simulink model "DSQPID"  (Simulink 7.8)
settings: Solver=ode4  StartTime=0.0  StopTime=2  FixedStep=0.001  RelTol=1e-3
settings Model: Creator=Zhu Supeng  LastModifiedBy=Zhu Supeng
settings DataIOCC: SignalLoggingName=sigsOut
settings DebuggingCC: SaveWithParameterizedLinksMsg=none  SignalResolutionControl=TryResolveAllWithWarning  SolverPrmCheckMsg=none  MultiTaskDSMMsg=warning  MultiTaskCondExecSysMsg=none  StrictBusMsg=None
settings HardwareCC: TargetUnknown=on
settings RTWCC: IncludeERTFirstTime=on

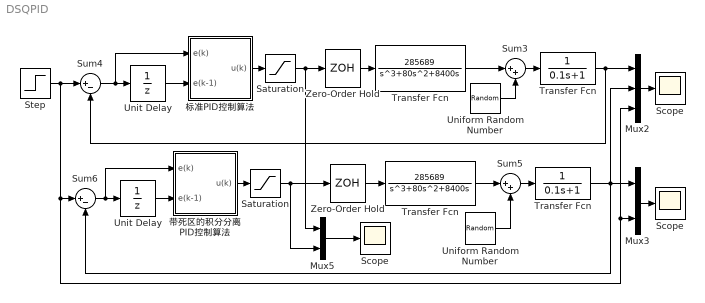
== system DSQPID ==
  "  Transfer Fcn " : TransferFcn  Denominator=[0.1 1]
  " Transfer Fcn " : TransferFcn  Denominator=[0.1 1]
  Mux2 : Mux  Inputs=3
  Mux3 : Mux  Inputs=2
  Mux5 : Mux  Inputs=2
  Saturation : Saturate  UpperLimit=10  LowerLimit=-10
  "Saturation " : Saturate  UpperLimit=10  LowerLimit=-10
  Scope : Scope
      settings: YMin=0.955  YMax=1.035  SaveName=DSQPIDy  DataFormat=Array  MaxDataPoints=500000
  "Scope " : Scope
      settings: YMin=-2  YMax=10  SaveName=DSQPIDu  DataFormat=Array  MaxDataPoints=500000
  "Scope  " : Scope
      settings: YMin=-0.2  YMax=1.2  SaveName=DSQPIDry  DataFormat=Array  MaxDataPoints=500000
  Step : Step  Time=0  SampleTime=0
  Sum3 : Sum  Inputs=|++  SaturateOnIntegerOverflow=on
  Sum4 : Sum  Inputs=|+-  SaturateOnIntegerOverflow=on
  Sum5 : Sum  Inputs=|++  SaturateOnIntegerOverflow=on
  Sum6 : Sum  Inputs=|+-  SaturateOnIntegerOverflow=on
  Transfer Fcn : TransferFcn  Numerator=[285689]  Denominator=[1 80 8400 0]
  "Transfer Fcn " : TransferFcn  Numerator=[285689]  Denominator=[1 80 8400 0]
  "Uniform Random Number " : UniformRandomNumber  Minimum=-0.5  Maximum=0.5  SampleTime=0
  "Uniform Random Number   " : UniformRandomNumber  Minimum=-0.5  Maximum=0.5  SampleTime=0
  Unit Delay : UnitDelay  SampleTime=0.001
  "Unit Delay " : UnitDelay  SampleTime=0.001
  Zero-Order Hold : ZeroOrderHold  SampleTime=0.001
  "Zero-Order Hold " : ZeroOrderHold  SampleTime=0.001
  带死区的积分分离 PID控制算法 : Subsystem
  标准PID控制算法 : Subsystem
  wires:
  "Transfer Fcn "/1 -> Sum5/1
  Sum5/1 -> " Transfer Fcn "/1
  "Uniform Random Number "/1 -> Sum5/2
  带死区的积分分离 PID控制算法/1(u(k)) -> "Saturation "/1
  "Unit Delay "/1 -> 带死区的积分分离 PID控制算法/2(e(k-1))
  Mux3/1 -> Scope/1
  " Transfer Fcn "/1 -> Mux3/1, Mux2/2, Sum6/2
  "Zero-Order Hold "/1 -> "Transfer Fcn "/1
  Mux5/1 -> "Scope "/1
  Step/1 -> Sum6/1, Mux2/3, Mux3/2, Sum4/1
  "Saturation "/1 -> "Zero-Order Hold "/1, Mux5/2
  Sum6/1 -> "Unit Delay "/1, 带死区的积分分离 PID控制算法/1(e(k))
  Transfer Fcn/1 -> Sum3/1
  Sum3/1 -> "  Transfer Fcn "/1
  标准PID控制算法/1(u(k)) -> Saturation/1
  Unit Delay/1 -> 标准PID控制算法/2(e(k-1))
  Sum4/1 -> 标准PID控制算法/1(e(k)), Unit Delay/1
  Mux2/1 -> "Scope  "/1
  Zero-Order Hold/1 -> Transfer Fcn/1
  Saturation/1 -> Zero-Order Hold/1, Mux5/1
  "  Transfer Fcn "/1 -> Sum4/2, Mux2/1
  "Uniform Random Number   "/1 -> Sum3/2

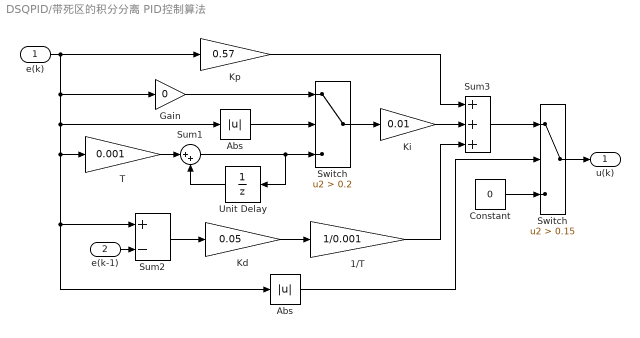
== system DSQPID/带死区的积分分离 PID控制算法 ==
  e(k) : Inport
  e(k-1) : Inport  Port=2
  1/T : Gain  Gain=1/0.001  SaturateOnIntegerOverflow=on  OutDataTypeStr=Inherit: Same as input  ParamDataTypeStr=Inherit: Same as input
  Abs : Abs  SaturateOnIntegerOverflow=on
  "Abs " : Abs  SaturateOnIntegerOverflow=on
  Constant : Constant  Value=0
  Gain : Gain  Gain=0  SaturateOnIntegerOverflow=on  OutDataTypeStr=Inherit: Same as input  ParamDataTypeStr=Inherit: Same as input
  Kd : Gain  Gain=0.05  SaturateOnIntegerOverflow=on  OutDataTypeStr=Inherit: Same as input  ParamDataTypeStr=Inherit: Same as input
  Ki : Gain  Gain=0.01  SaturateOnIntegerOverflow=on  OutDataTypeStr=Inherit: Same as input  ParamDataTypeStr=Inherit: Same as input
  Kp : Gain  Gain=0.57  SaturateOnIntegerOverflow=on  OutDataTypeStr=Inherit: Same as input  ParamDataTypeStr=Inherit: Same as input
  Sum1 : Sum  Inputs=|++  SaturateOnIntegerOverflow=on
  Sum2 : Sum  Inputs=+-  SaturateOnIntegerOverflow=on
  Sum3 : Sum  Inputs=+++  SaturateOnIntegerOverflow=on
  Switch : Switch  Criteria=u2 > Threshold  Threshold=0.2  SaturateOnIntegerOverflow=on  InputSameDT=on
  "Switch " : Switch  Criteria=u2 > Threshold  Threshold=0.15  SaturateOnIntegerOverflow=on  InputSameDT=on
  T : Gain  Gain=0.001  SaturateOnIntegerOverflow=on  OutDataTypeStr=Inherit: Same as input  ParamDataTypeStr=Inherit: Same as input
  "Unit Delay " : UnitDelay  SampleTime=0.001
  u(k) : Outport
  wires:
  Sum3/1 -> "Switch "/1
  Ki/1 -> Sum3/2
  1/T/1 -> Sum3/3
  e(k-1)/1 -> Sum2/2
  Kd/1 -> 1/T/1
  Kp/1 -> Sum3/1
  e(k)/1 -> Kp/1, Gain/1, Abs/1, T/1, Sum2/1, "Abs "/1
  Sum2/1 -> Kd/1
  T/1 -> Sum1/1
  "Unit Delay "/1 -> Sum1/2
  Sum1/1 -> "Unit Delay "/1, Switch/3
  "Abs "/1 -> "Switch "/2
  Constant/1 -> "Switch "/3
  "Switch "/1 -> u(k)/1
  Switch/1 -> Ki/1
  Gain/1 -> Switch/1
  Abs/1 -> Switch/2

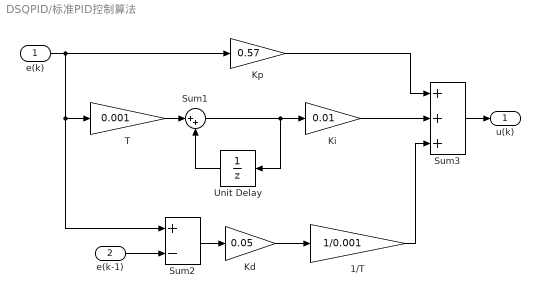
== system DSQPID/标准PID控制算法 ==
  e(k) : Inport
  e(k-1) : Inport  Port=2
  1/T : Gain  Gain=1/0.001  SaturateOnIntegerOverflow=on  OutDataTypeStr=Inherit: Same as input  ParamDataTypeStr=Inherit: Same as input
  Kd : Gain  Gain=0.05  SaturateOnIntegerOverflow=on  OutDataTypeStr=Inherit: Same as input  ParamDataTypeStr=Inherit: Same as input
  Ki : Gain  Gain=0.01  SaturateOnIntegerOverflow=on  OutDataTypeStr=Inherit: Same as input  ParamDataTypeStr=Inherit: Same as input
  Kp : Gain  Gain=0.57  SaturateOnIntegerOverflow=on  OutDataTypeStr=Inherit: Same as input  ParamDataTypeStr=Inherit: Same as input
  Sum1 : Sum  Inputs=|++  SaturateOnIntegerOverflow=on
  Sum2 : Sum  Inputs=+-  SaturateOnIntegerOverflow=on
  Sum3 : Sum  Inputs=+++  SaturateOnIntegerOverflow=on
  T : Gain  Gain=0.001  SaturateOnIntegerOverflow=on  OutDataTypeStr=Inherit: Same as input  ParamDataTypeStr=Inherit: Same as input
  Unit Delay : UnitDelay  SampleTime=0.001
  u(k) : Outport
  wires:
  Sum3/1 -> u(k)/1
  Ki/1 -> Sum3/2
  1/T/1 -> Sum3/3
  e(k-1)/1 -> Sum2/2
  Kd/1 -> 1/T/1
  Kp/1 -> Sum3/1
  e(k)/1 -> Kp/1, Sum2/1, T/1
  Sum2/1 -> Kd/1
  T/1 -> Sum1/1
  Unit Delay/1 -> Sum1/2
  Sum1/1 -> Unit Delay/1, Ki/1
